simulink subsystem "duffing"  (R2019b)
settings: Solver=FixedStepAuto  StartTime=0.0  StopTime=10.0  FixedStep=dt  RelTol=1e-3
undefined symbols (not defined in the file): beta, delta, gamma, omega, omega2, phi, x0
settings Model: Creator=enrique.babio  LastModifiedBy=enrique.babio

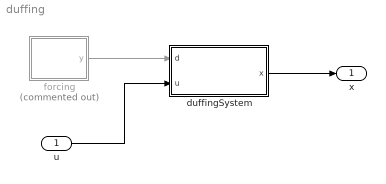
== system duffing ==
  u : Inport  OutDataTypeStr=double  PortDimensions=1  SampleTime=0
  duffingSystem : Subsystem
  forcing : Subsystem  Commented=on
  x : Outport  OutDataTypeStr=double  SampleTime=0
  wires:
  duffingSystem/1(x) -> x/1
  u/1 -> duffingSystem/2(u)
  forcing/1(y) -> duffingSystem/1(d)

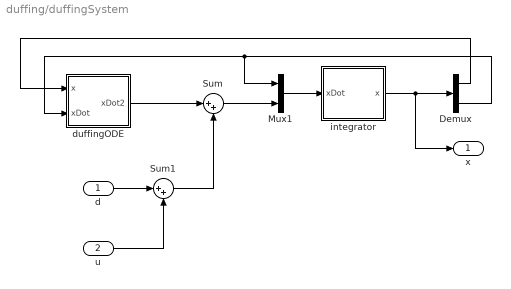
== system duffing/duffingSystem ==
  d : Inport
  u : Inport  Port=2
  Demux : Demux  Outputs=2
  Mux1 : Mux  Inputs=2
  Sum : Sum  Inputs=|++
  Sum1 : Sum  Inputs=|++
  duffingODE : Subsystem
  integrator : Subsystem
  x : Outport
  wires:
  Demux/2 -> duffingODE/2(xDot), Mux1/1
  Demux/1 -> duffingODE/1(x)
  integrator/1(x) -> Demux/1, x/1
  Mux1/1 -> integrator/1(xDot)
  Sum/1 -> Mux1/2
  duffingODE/1(xDot2) -> Sum/1
  d/1 -> Sum1/1
  Sum1/1 -> Sum/2
  u/1 -> Sum1/2

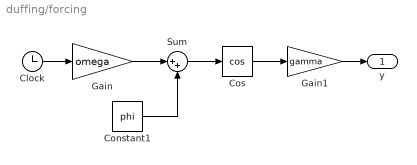
== system duffing/forcing ==
  Clock : Clock
  Constant1 : Constant  Value=phi
  Cos : Trigonometry  Operator=cos
  Gain : Gain  Gain=omega
  Gain1 : Gain  Gain=gamma
  Sum : Sum  Inputs=|++
  y : Outport
  wires:
  Sum/1 -> Cos/1
  Clock/1 -> Gain/1
  Gain/1 -> Sum/1
  Cos/1 -> Gain1/1
  Constant1/1 -> Sum/2
  Gain1/1 -> y/1

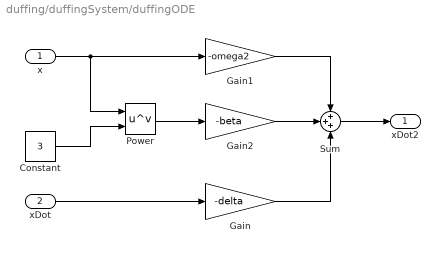
== system duffing/duffingSystem/duffingODE ==
  x : Inport
  xDot : Inport  Port=2
  Constant : Constant  Value=3
  Gain : Gain  Gain=-delta
  Gain1 : Gain  Gain=-omega2
  Gain2 : Gain  Gain=-beta
  Power : Math  Operator=pow  SignedPower=off  SaturateOnIntegerOverflow=on
  Sum : Sum  Inputs=+++
  xDot2 : Outport
  wires:
  x/1 -> Power/1, Gain1/1
  xDot/1 -> Gain/1
  Constant/1 -> Power/2
  Power/1 -> Gain2/1
  Sum/1 -> xDot2/1
  Gain1/1 -> Sum/1
  Gain2/1 -> Sum/2
  Gain/1 -> Sum/3

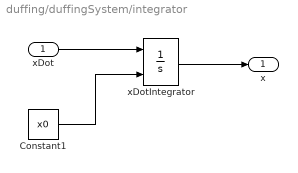
== system duffing/duffingSystem/integrator ==
  xDot : Inport
  Constant1 : Constant  Value=x0
  xDotIntegrator : Integrator  InitialConditionSource=external  InitialCondition=x0(2)  ContinuousStateAttributes='x'
  x : Outport
  wires:
  xDot/1 -> xDotIntegrator/1
  xDotIntegrator/1 -> x/1
  Constant1/1 -> xDotIntegrator/2
